simulink model "control_dynamic_no_vel"  (R2020a)
settings: Solver=ode3  StartTime=0.0  StopTime=10.0  RelTol=1e-3
libraries: roblocks x4
settings Model: Creator=robot  LastModifiedBy=robot

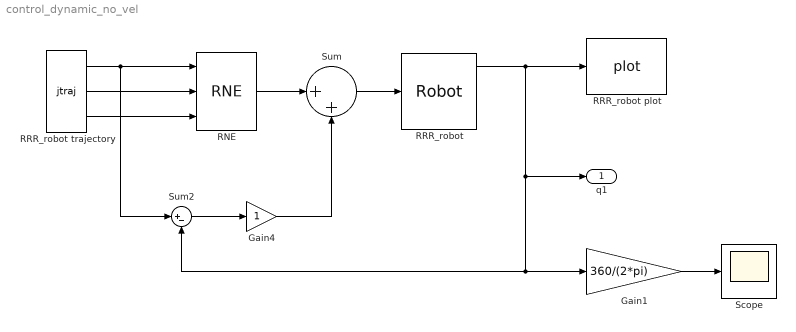
== system control_dynamic_no_vel ==
  Gain1 : Gain  Gain=360/(2*pi)
  Gain4 : Gain
  RNE : roblocks/Arm/RNE  robot=RRR_robot  grav=[0 0 9.81]
  RRR_robot : roblocks/Arm/Robot  robot=RRR_robot  q0=[0 0 0]
  RRR_robot plot : roblocks/Arm/plot  robot=RRR_robot  fps=5  holdplot=on
  RRR_robot trajectory : roblocks/Toolbox/jtraj  q0=[0 0 0]  qf=[pi/2 -pi/4 -pi/4]  tmax=2  ts=0.02
  Scope : Scope
  Sum : Sum  Inputs=|++
  Sum2 : Sum  Inputs=|+-
  q1 : Outport
  wires:
  Sum2/1 -> Gain4/1
  RRR_robot trajectory/1 -> Sum2/1, RNE/1
  Sum/1 -> RRR_robot/1
  RRR_robot trajectory/2 -> RNE/2
  Gain1/1 -> Scope/1
  RRR_robot/1 -> RRR_robot plot/1, q1/1, Gain1/1, Sum2/2
  RRR_robot trajectory/3 -> RNE/3
  RNE/1 -> Sum/1
  Gain4/1 -> Sum/2
